simulink model "ValidacionSimulink"  (R2022b)
settings: Solver=VariableStepAuto  StartTime=0.0  StopTime=10  RelTol=1e-3
values from neighbouring files (symbols this model uses):
  tt = tr-tr(1)    [LAB.m]
  ut = ur-u(pos(1)-1)    [LAB.m]
settings Model: Creator=emanu  LastModifiedBy=emanu

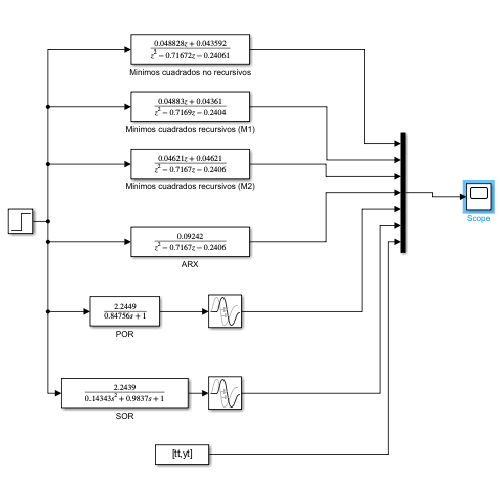
[thumbnail: Simulink's stored preview of the top-level diagram]
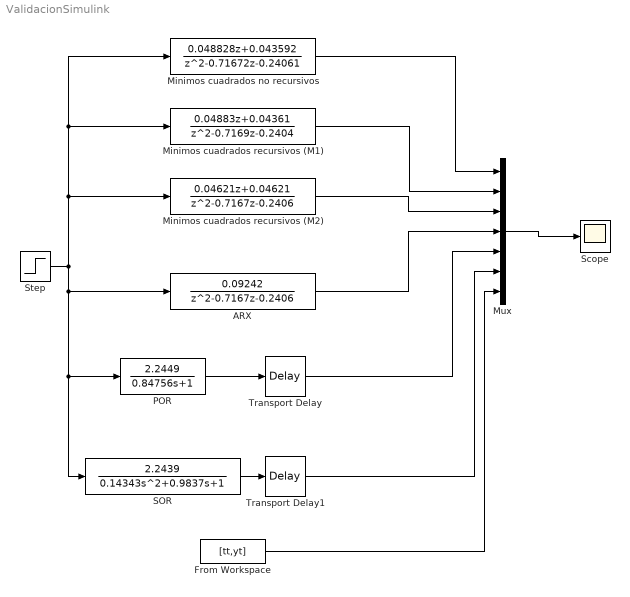
== system ValidacionSimulink ==
  ARX : DiscreteTransferFcn  Numerator=[0 0.09242]  Denominator=[1 -0.7167 -0.2406]  SampleTime=tt(2)
  From Workspace : FromWorkspace  VariableName=[tt,yt]  SampleTime=tt(2)
  Minimos cuadrados no recursivos : DiscreteTransferFcn  Numerator=[0 0.048828 0.043592]  Denominator=[1 -0.71672 -0.24061]  SampleTime=tt(2)
  Minimos cuadrados recursivos (M1) : DiscreteTransferFcn  Numerator=[0 0.04883 0.04361]  Denominator=[1 -0.7169 -0.2404]  SampleTime=tt(2)
  Minimos cuadrados recursivos (M2) : DiscreteTransferFcn  Numerator=[0 0.04621 0.04621]  Denominator=[1 -0.7167 -0.2406]  SampleTime=tt(2)
  Mux : Mux  Inputs=7
  POR : TransferFcn  Numerator=[2.2449]  Denominator=[0.84756 1]
  SOR : TransferFcn  Numerator=[2.2439]  Denominator=[0.14343 0.9837 1]
  Scope : Scope
  Step : Step  Time=0  After=ut(1)  SampleTime=0
  Transport Delay : TransportDelay  DelayTime=0.35428
  Transport Delay1 : TransportDelay  DelayTime=0.19318
  wires:
  POR/1 -> Transport Delay/1
  SOR/1 -> Transport Delay1/1
  Step/1 -> POR/1, SOR/1, ARX/1, Minimos cuadrados recursivos (M2)/1, Minimos cuadrados recursivos (M1)/1, Minimos cuadrados no recursivos/1
  Transport Delay1/1 -> Mux/6
  Transport Delay/1 -> Mux/5
  ARX/1 -> Mux/4
  Minimos cuadrados recursivos (M2)/1 -> Mux/3
  Minimos cuadrados recursivos (M1)/1 -> Mux/2
  Minimos cuadrados no recursivos/1 -> Mux/1
  Mux/1 -> Scope/1
  From Workspace/1 -> Mux/7
